simulink model "a_20210426_ahrs"  (R2020b)
settings: Solver=FixedStepDiscrete  StartTime=0.0  StopTime=inf  FixedStep=0.02  RelTol=1e-3  EnableMultiTasking=on
libraries: svdutilitieslib x2, arduinolib x1
settings Model: SILPILModeSetting=veronly  ExtModeTrigDuration=2  Creator=ricca  LastModifiedBy=ricca
settings OptimizationCC: EnhancedBackFolding=on  PassReuseOutputArgsAs=Individual arguments  ZeroExternalMemoryAtStartup=off  ZeroInternalMemoryAtStartup=off  MaxStackSize=64  OptimizeBlockOrder=speed  DifferentSizesBufferReuse=on  OptimizationCustomize=off  EfficientTunableParamExpr=on
settings DebuggingCC: ParameterTunabilityLossMsg=error
settings HardwareCC: ProdBitPerPointer=32  ProdBitPerSizeT=32  ProdBitPerPtrDiffT=32  ProdLargestAtomicInteger=Long  ProdLargestAtomicFloat=Double  ProdWordSize=32  ProdHWDeviceType=ARM Compatible->ARM Cortex
settings SFSimCC: MATLABDynamicMemAlloc=off
settings RTWCC: Description=Embedded Coder  SystemTargetFile=ert.tlc  HardwareBoard=Arduino Due  TemplateMakefile=ert_default_tmf  Toolchain=Arduino ARM  BuildConfiguration=Faster Runs
settings CodeAppCC: ForceParamTrailComments=on  IgnoreCustomStorageClasses=off  OperatorAnnotations=on  SimulinkDataObjDesc=on  SFDataObjDesc=on  InsertBlockDesc=on
settings ERTTargetCC: SupportContinuousTime=on  SupportVariableSizeSignals=on  ExtModeTransport=3  ExtModeStaticAllocSize=24576  ExtModeMexFile=ext_xcp  ExtModeIntrfLevel=Level2 - Open

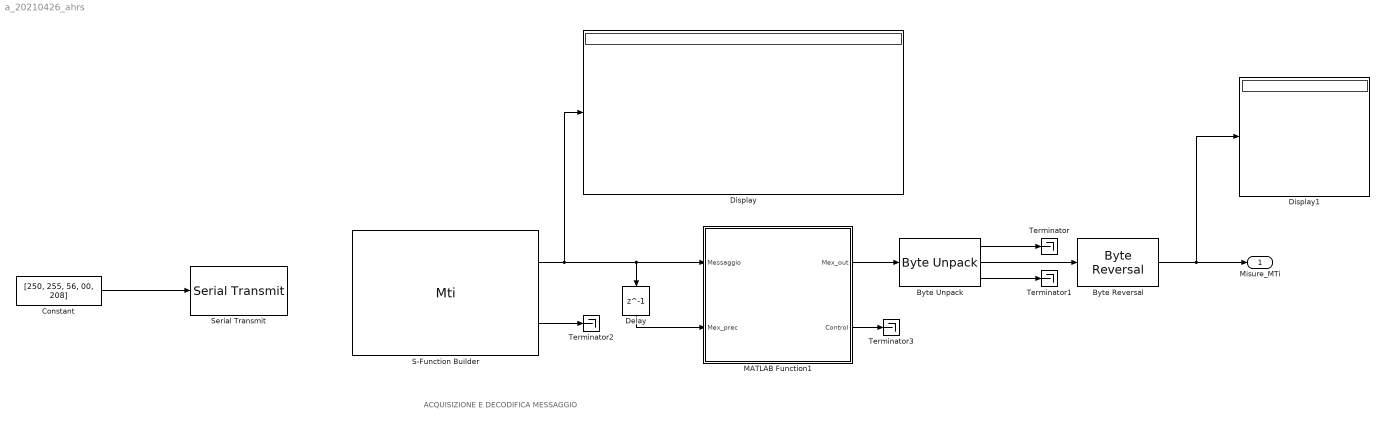
== system a_20210426_ahrs ==
  note: ACQUISIZIONE E DECODIFICA MESSAGGIO
  Byte Reversal : svdutilitieslib/Byte Reversal  numInp=1  blockPlatform=arduinoert
      settings: SourceProductBaseCode=ANDROID,ARDUINO,ML_ARDUINO,ECCORTEXA,ECCORTEXR,SC_BEAGLEBONE_BLUE,EC_FREEDOM_BOARD,EC_FRDM_K64F,INTEL_BLOCKSET,JETSONCPU,MICROBIT,NUCLEO,NVIDIA,PX4AUTOPILOTS,RASPPIIO,STMICRODIS,TIC2000,XILINX_BLOCKSET
  Byte Unpack : svdutilitieslib/Byte Unpack  dimensions={[4],[9],[1]}  datatypes={'uint8','single','uint8'}  byteAlign=1  blockPlatform=arduinoert
      settings: SourceProductBaseCode=ANDROID,ARDUINO,ML_ARDUINO,ECCORTEXA,ECCORTEXR,SC_BEAGLEBONE_BLUE,EC_FREEDOM_BOARD,EC_FRDM_K64F,INTEL_BLOCKSET,JETSONCPU,MICROBIT,NUCLEO,NVIDIA,PX4AUTOPILOTS,RASPPIIO,STMICRODIS,TIC2000,XILINX_BLOCKSET
  Constant : Constant  Value=[250, 255, 56, 00, 208]  OutDataTypeStr=uint8  SampleTime=0.02
  Delay : Delay  DelayLength=1
  Display : Display
  Display1 : Display
  MATLAB Function1 : MATLAB Function  TreatAsAtomicUnit=on
  S-Function Builder : S-Function  InitFcn=try, set_param(gcb,'FunctionName','Mti'), end  FunctionName=Mti  SFunctionModules=Mti_wrapper  SFunctionDeploymentMode=off  EnableBusSupport=off  mask(S-Function Builder){}
      mask help: Simulink:masks:SFunctionBuilder_MD
      mask init:
      | val = [[.9  0.75 0.75 1 1 .9 .9 1]',[1 1 0.75 0.75 .9 .9 1 .9]'];try , sys = get_param(gcb,'SfunBuilderFcnName');if isempty(sys), sys = get_param(gcb,'FunctionName'); end,catch, sys = get_param(gcb,'FunctionName'); end
      settings: CopyFcn=set_param(gcbh,'LinkStatus','none')  PreSaveFcn=try, set_param(gcb,'FunctionName','Mti'), end  OpenFcn=sfunctionwizard(gcbh)
      mask Display:
      | plot(val(:,1),val(:,2))
      | disp(sys)
      | port_label('output',1,'Messaggio')
      | port_label('output',2,'Control')
  Serial Transmit : arduinolib/Serial Transmit  portNumber=3  sendmode=write  sendformat=Decimal  floatprecision=2  blockPlatform=arduino
  Terminator{,1..3} (4 alike) : Terminator
  Misure_MTi : Outport  VectorParamsAs1DForOutWhenUnconnected=off
  wires:
  Delay/1 -> MATLAB Function1/2(Mex_prec)
  MATLAB Function1/1(Mex_out) -> Byte Unpack/1
  S-Function Builder/1 -> Delay/1, MATLAB Function1/1(Messaggio), Display/1
  S-Function Builder/2 -> Terminator2/1
  MATLAB Function1/2(Control) -> Terminator3/1
  Byte Unpack/2 -> Byte Reversal/1
  Byte Unpack/3 -> Terminator1/1
  Byte Reversal/1 -> Display1/1, Misure_MTi/1
  Byte Unpack/1 -> Terminator/1
  Constant/1 -> Serial Transmit/1

== matlab function a_20210426_ahrs/MATLAB Function1 ==
  data: Messaggio input; Mex_out output; Mex_prec input; Control output
function [Mex_out,Control]  = checksum_control(Messaggio,Mex_prec)

Control = uint8(0);

mti_string = uint8(Messaggio(2:41));

checksum = sum(mti_string) ; 

hex_checksum = dec2hex(checksum);

if ((hex_checksum(3) == '0') && (hex_checksum(4) == '0'))
    Mex_out = uint8(Messaggio);

else
   Control = uint8(1); 
   Mex_out = Mex_prec;   
end



end
